simulink model "threeDiskOscillatorRig_Q6_experiment"  (R2020a)
settings: Solver=VariableStepAuto  StartTime=0.0  StopTime=simTime  RelTol=1e-8
values from neighbouring files (symbols this model uses):
  h = 7.56835261331    [ECP_state_space.mat]    (also in threeDiskOscillator_ALL.m = chi2inv(1 - P_F, 1)/2)
  M = 64    [ECP_state_space.mat]    (also in threeDiskOscillator_ALL.m = ceil(double(vpasolve([integral == P_D], [M], [0 200]))))
  mu_0 = 0    [ECP_state_space.mat]    (also in threeDiskOscillator_ALL.m)
  r_window = [0 0 0 0 0 0 0 0 0 0 0 0 ... (64 elements, 64x1)]    [ECP_state_space.mat]    (also in threeDiskOscillator_ALL.m = zeros(M,1))
  sigma_yr = 44.3946006619    [ECP_state_space.mat]    (also in threeDiskOscillator_ALL.m = sqrt(Q_yr))
  T_s = 0.004    [ECP_state_space.mat]    (also in threeDiskOscillator_ALL.m)
settings Model: Creator=dimpa  LastModifiedBy=Administrator
settings DataIOCC: ReturnWorkspaceOutputs=off
settings DebuggingCC: ArithmeticOperatorsInVariantConditions=warning
settings SFSimCC: SimUseLocalCustomCode=off  CustomCodeUndefinedFunction=UseInterfaceOnly
settings RTWCC: RTWUseLocalCustomCode=off

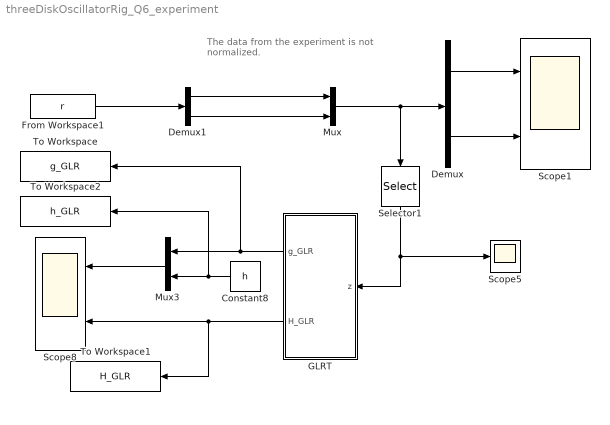
== system threeDiskOscillatorRig_Q6_experiment ==
  note: The data from the experiment is not
      | normalized.
  Constant8 : Constant  Value=h
  Demux : Demux  Outputs=2
  Demux1 : Demux  Outputs=2
  From Workspace1 : FromWorkspace  VariableName=r  SampleTime=T_s
  GLRT : Subsystem
  Mux : Mux  Inputs=2
  Mux3 : Mux  Inputs=2
  Scope1 : Scope  NumInputPorts=2
  Scope5 : Scope
  Scope8 : Scope  NumInputPorts=2
  Selector1 : Selector  InputPortWidth=2  IndexOptions=Index vector (dialog)  Indices=[2]  OutputSizes=1
  To Workspace : ToWorkspace  VariableName=g_GLR  SaveFormat=Timeseries  SampleTime=-1
  To Workspace1 : ToWorkspace  VariableName=H_GLR  SaveFormat=Timeseries  SampleTime=T_s
  To Workspace2 : ToWorkspace  VariableName=h_GLR  SaveFormat=Timeseries  SampleTime=T_s
  wires:
  GLRT/1(g_GLR) -> To Workspace/1, Mux3/1
  GLRT/2(H_GLR) -> To Workspace1/1, Scope8/2
  Constant8/1 -> To Workspace2/1, Mux3/2
  Mux3/1 -> Scope8/1
  Demux/1 -> Scope1/1
  Demux/2 -> Scope1/2
  Selector1/1 -> Scope5/1, GLRT/1(z)
  From Workspace1/1 -> Demux1/1
  Demux1/1 -> Mux/1
  Mux/1 -> Selector1/1, Demux/1
  Demux1/2 -> Mux/2

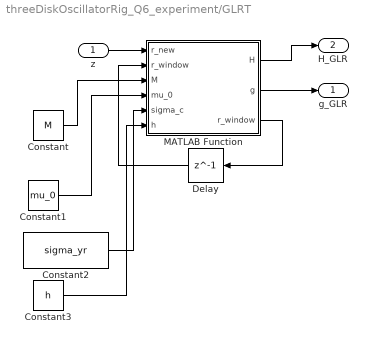
== system threeDiskOscillatorRig_Q6_experiment/GLRT ==
  z : Inport
  Constant : Constant  Value=M
  Constant1 : Constant  Value=mu_0
  Constant2 : Constant  Value=sigma_yr
  Constant3 : Constant  Value=h
  Delay : Delay  DelayLength=1  InitialCondition=r_window  SampleTime=T_s
  MATLAB Function : MATLAB Function  TreatAsAtomicUnit=on
  g_GLR : Outport  VectorParamsAs1DForOutWhenUnconnected=off
  H_GLR : Outport  Port=2  VectorParamsAs1DForOutWhenUnconnected=off
  wires:
  z/1 -> MATLAB Function/1(r_new)
  MATLAB Function/3(r_window) -> Delay/1
  MATLAB Function/2(g) -> g_GLR/1
  MATLAB Function/1(H) -> H_GLR/1
  Delay/1 -> MATLAB Function/2("r_window ")
  Constant2/1 -> MATLAB Function/5(sigma_c)
  Constant1/1 -> MATLAB Function/4(mu_0)
  Constant/1 -> MATLAB Function/3(M)
  Constant3/1 -> MATLAB Function/6(h)

== matlab function threeDiskOscillatorRig_Q6_experiment/GLRT/MATLAB Function ==
  data: r_new input; H output; r_window input; g output; r_window output; M input; mu_0 input; sigma_c input; h input
function [H, g, r_window] = GLR(r_new, r_window, M, mu_0, sigma_c, h)

%sigma = 0.36229693539067544172329302373852;
%mu_0 = 0;
%M = 265;
%h=7.5684;

r_window = [r_window(2:end); r_new];


%Using equation 7.35 from the book

%calculating g from a running window.
g = 1/(2*sigma_c^2*M)*(sum(r_window-mu_0))^2;

if (g > h)
    H = 1;
else
    H = 0;
end
